simulink model "neural_net_model"  (R2021a)
settings: Solver=FixedStepAuto  StartTime=0.0  StopTime=inf  FixedStep=0.05  RelTol=1e-3
libraries: robotlib x4, deeplib x1
settings Model: Creator=refulgent  LastModifiedBy=refulgent
settings OptimizationCC: EnhancedBackFolding=on  PassReuseOutputArgsAs=Individual arguments  ZeroExternalMemoryAtStartup=off  ZeroInternalMemoryAtStartup=off  MaxStackSize=64  OptimizeBlockOrder=speed  DifferentSizesBufferReuse=on  OptimizationCustomize=off  EfficientTunableParamExpr=on
settings DebuggingCC: ParameterTunabilityLossMsg=error
settings HardwareCC: ProdBitPerPointer=32  ProdBitPerSizeT=32  ProdBitPerPtrDiffT=32  ProdLargestAtomicFloat=None  ProdIntDivRoundTo=Undefined  ProdEndianess=Unspecified  ProdWordSize=32  ProdHWDeviceType=Generic->Unspecified (assume 32-bit Generic)
settings SFSimCC: MATLABDynamicMemAlloc=off
settings RTWCC: SystemTargetFile=ert.tlc  HardwareBoard=Robot Operating System (ROS)  TLCOptions="-aInlineSetEventsForThisBaseRateFcn=TLC_FALSE -aSuppressMultiTaskScheduler=TLC_FALSE  -aRateBasedStepFcn=0"  TemplateMakefile=ert_default_tmf  GenerateReport=on  Toolchain=Catkin  LaunchReport=on  TargetLang=C++  GenerateWebview=on
settings CodeAppCC: ForceParamTrailComments=on  IgnoreCustomStorageClasses=off  OperatorAnnotations=on  SimulinkDataObjDesc=on  SFDataObjDesc=on  InsertBlockDesc=on

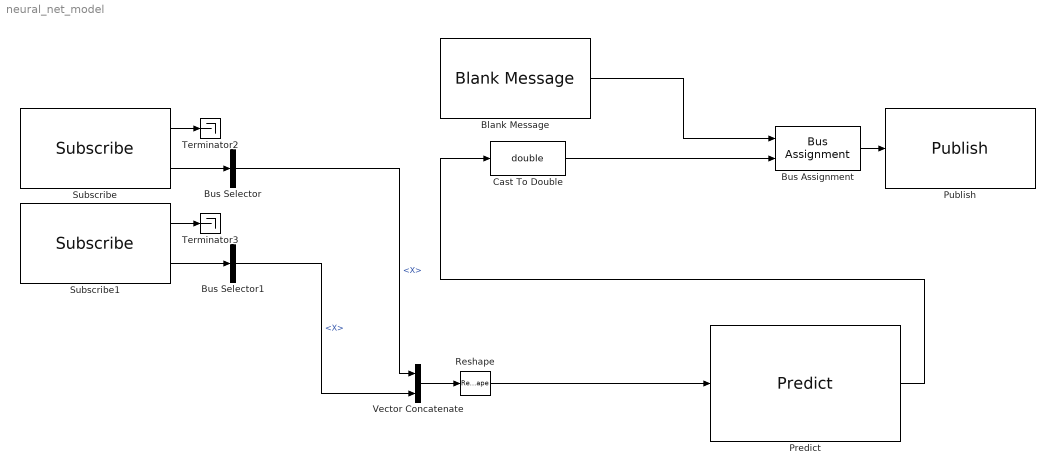
== system neural_net_model ==
  Blank Message : robotlib/Blank Message  messageClass=Message  entityType=geometry_msgs/Twist  messageType=geometry_msgs/Twist  SampleTime=inf  legacyBusStruct=off
  Bus Assignment : BusAssignment  AssignedSignals=Linear.X
  Bus Selector : BusSelector  OutputSignals=Linear.X
  Bus Selector1 : BusSelector  OutputSignals=Linear.X
  Cast To Double : DataTypeConversion  OutDataTypeStr=double
  Predict : deeplib/Predict  Network=Network from MAT-file  NetworkFunction=squeezenet  NetworkFilePath=/home/refulgent/VersionControl/medium.com/01_12_2021/net.mat  MiniBatchSize=128  InputDataFormats={ '', '' }  Predictions=on  Activations={}  ForceInterpretedSim=off  EnableDLNetwork=on
      settings: SourceProductBaseCode=NN
  Publish : robotlib/Publish  topicSource=Specify your own  topic=accel  messageType=geometry_msgs/Twist  legacyBusStruct=off  messageQueueLength=1
  Reshape : Reshape  OutputDimensionality=Row vector (2-D)
  Subscribe : robotlib/Subscribe  topicSource=Specify your own  topic=cmd_vel  messageType=geometry_msgs/Twist  SampleTime=-1  legacyBusStruct=off  messageQueueLength=1
  Subscribe1 : robotlib/Subscribe  topicSource=Specify your own  topic=yaw_rate  messageType=geometry_msgs/Twist  SampleTime=-1  legacyBusStruct=off  messageQueueLength=1
  Terminator2 : Terminator
  Terminator3 : Terminator
  Vector Concatenate : Concatenate
  wires:
  Reshape/1 -> Predict/1
  Vector Concatenate/1 -> Reshape/1
  Subscribe/2 -> Bus Selector/1
  Bus Selector1/1 -> Vector Concatenate/2  "<X>"
  Bus Selector/1 -> Vector Concatenate/1  "<X>"
  Subscribe1/2 -> Bus Selector1/1
  Subscribe/1 -> Terminator2/1
  Subscribe1/1 -> Terminator3/1
  Predict/1 -> Cast To Double/1
  Blank Message/1 -> Bus Assignment/1
  Bus Assignment/1 -> Publish/1
  Cast To Double/1 -> Bus Assignment/2
